simulink model "OLD_bidirection_buck_boost"  (R2025a)
settings: Solver=VariableStepAuto  StartTime=0.0  StopTime=0.1  MaxStep=1e-7  RelTol=1e-3
libraries: spsMosfetLib x5, spsPWMGeneratorDCDCLib x4, spsSeriesRLCBranchLib x4, spsCurrentMeasurementLib x3, spsVoltageMeasurementLib x2, spsDCVoltageSourceLib x1, spsGroundLib x1, spsMeanLib x1, spsPVArrayLib x1, spspowerguiLib x1
settings Model: Creator=GNKRISHNAN  LastModifiedBy=GNKRISHNAN

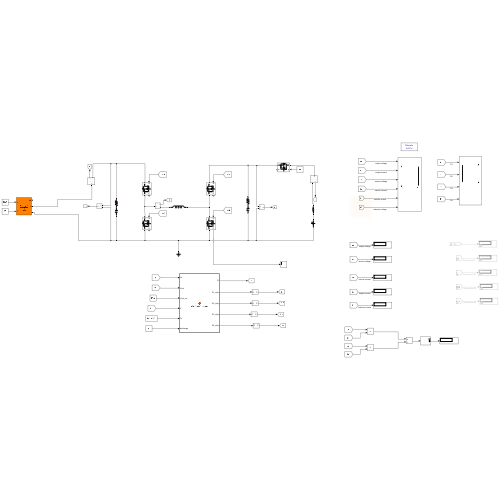
[thumbnail: Simulink's stored preview of the top-level diagram]
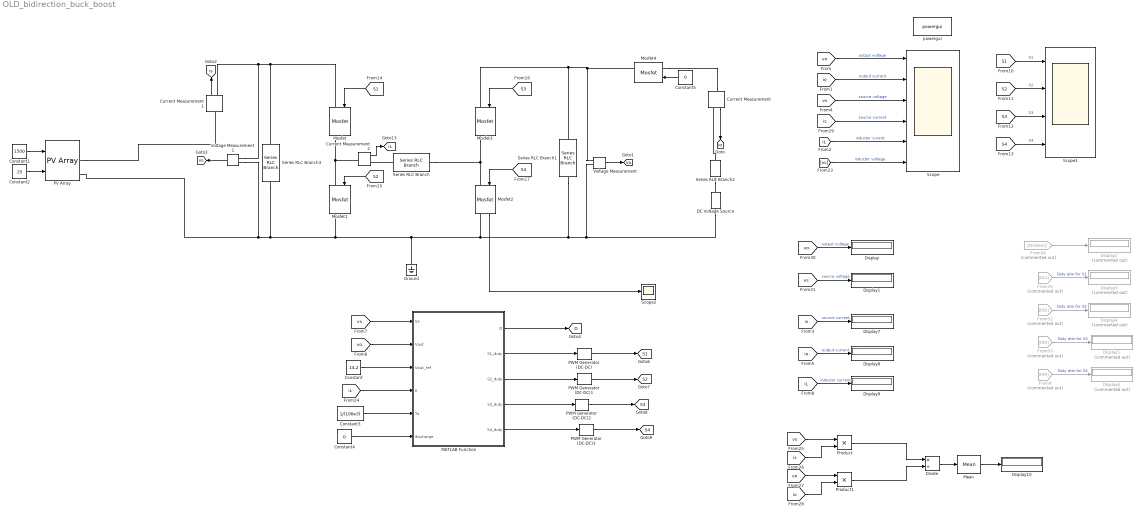
== system OLD_bidirection_buck_boost ==
  Constant : Constant  Value=14.2
  Constant1 : Constant  Value=1500
  Constant2 : Constant  Value=25
  Constant3 : Constant  Value=1/(100e3)
  Constant4 : Constant  Value=0
  Constant5 : Constant  Value=0
  Current Measurement : spsCurrentMeasurementLib/Current Measurement  PhasorSimulation=off  OutputType=Complex  PSBequivalent=0
  Current Measurement1 : spsCurrentMeasurementLib/Current Measurement  PhasorSimulation=off  OutputType=Complex  PSBequivalent=0
  Current Measurement2 : spsCurrentMeasurementLib/Current Measurement  PhasorSimulation=off  OutputType=Complex  PSBequivalent=0
  DC Voltage Source : spsDCVoltageSourceLib/DC Voltage Source  Amplitude=12  Measurements=None
  Display{,1,7..10} (6 alike) : Display
  Display{2..6} (5 alike) : Display  Commented=on
  Divide : Product  Inputs=*/
  From32 : From  Commented=on  GotoTag=DS2  TagVisibility=global
  From33 : From  Commented=on  GotoTag=DS3  TagVisibility=global
  From34 : From  Commented=on  GotoTag=Dintern  TagVisibility=global
  From35 : From  Commented=on  GotoTag=DS1  TagVisibility=global
  From9 : From  Commented=on  GotoTag=DS4  TagVisibility=global
  Ground : spsGroundLib/Ground  LConnTagsString=a
  MATLAB Function : MATLAB Function  TreatAsAtomicUnit=on  SystemSampleTime=1/(100e3)
  Mean : spsMeanLib/Mean  Freq=1/100e3  Vinit=0  Ts=0
  Mosfet{,1..3} (4 alike) : spsMosfetLib/Mosfet  Ron=0.1  Lon=0  Rd=0.0028  Vfd=0.7  IC=0  Rs=1e5  Cs=inf  Measurements=on
  Mosfet4 : spsMosfetLib/Mosfet  Ron=0.1  Lon=0  Rd=0.01  Vfd=0  IC=0  Rs=1e5  Cs=inf  Measurements=on
  PV Array : spsPVArrayLib/PV Array  Npar=1  Nser=1  PlotType=one module @ 25 deg.C & specified irradiances  S_vec="[ 1000  500  100 ]"  Temp_C_vec="[ 45 25  ]"  ModuleName=GCL System Integration Technology Co._ Ltd. GCL-P6/72355  PlotWhenSelected=off  Pm=355.0151  Ncell=72  Voc=47.9  Isc=9.74  Vm=39.49  Im=8.99  beta_Voc_pc=-0.296  alpha_Isc_pc=0.041201  beta_Voc=-0.14178  alpha_Isc=0.004013  IL=9.7653  I0=2.744e-11  nI=0.97505  Rsh=121.7675  Rs=0.31609  RobustModel=off  RobustCellTemperature=313.3991  BAL=on  Tc=1e-6  Tfilter=5e-5
  PWM Generator (DC-DC){,1..3} (4 alike) : spsPWMGeneratorDCDCLib/PWM Generator (DC-DC)  Fsw=100e3  Ts=0
  Product : Product
  Product1 : Product
  Scope : Scope  NumInputPorts=6
      settings: ActiveDisplayYMinimum=-1.5008435166057172  ActiveDisplayYMaximum=13.509037415165276
  Scope1 : Scope  NumInputPorts=4
      settings: ActiveDisplayYMinimum=-0.12499999999999997  ActiveDisplayYMaximum=1.125
  Scope2 : Scope
      settings: ActiveDisplayYMinimum=-1.430223431644835  ActiveDisplayYMaximum=12.872010884803517  DataLoggingVariableName=ScopeData2
  Series RLC Branch : spsSeriesRLCBranchLib/Series RLC Branch  LConnTagsString=__new0  RConnTagsString=__new0  BranchType=L  Resistance=0.001  Inductance=150e-6  SetiL0=on  InitialCurrent=0  Capacitance=1e-6  Setx0=off  InitialVoltage=0  Measurements=None
  Series RLC Branch1 : spsSeriesRLCBranchLib/Series RLC Branch  LConnTagsString=__new0  RConnTagsString=__new0  BranchType=RC  Resistance=0.0001  Inductance=1e-3  SetiL0=off  InitialCurrent=0  Capacitance=100e-6  Setx0=on  InitialVoltage=0  Measurements=None
  Series RLC Branch2 : spsSeriesRLCBranchLib/Series RLC Branch  LConnTagsString=__new0  RConnTagsString=__new0  BranchType=R  Resistance=83e-3  Inductance=1e-3  SetiL0=off  InitialCurrent=0  Capacitance=1e-6  Setx0=off  InitialVoltage=0  Measurements=None
  Series RLC Branch3 : spsSeriesRLCBranchLib/Series RLC Branch  LConnTagsString=__new0  RConnTagsString=__new0  BranchType=RC  Resistance=0.0001  Inductance=1e-3  SetiL0=off  InitialCurrent=0  Capacitance=100e-6  Setx0=on  InitialVoltage=0  Measurements=None
  Voltage Measurement : spsVoltageMeasurementLib/Voltage Measurement  PhasorSimulation=off  OutputType=Complex  PSBequivalent=0
  Voltage Measurement1 : spsVoltageMeasurementLib/Voltage Measurement  PhasorSimulation=off  OutputType=Complex  PSBequivalent=0
  powergui : spspowerguiLib/powergui  Priority=1  SimulationMode=Discrete  SampleTime=1e-7  frequency=60  Iterations=50  frequencyindice=0  Pbase=100e6  ErrMax=1e-4  UnitsV=kV  UnitsW=MW  buscounter=0  FunctionMessages=off  echomessages=off  EnableUseOfTLC=off  CurrentSourceSwitches=off  DisableSnubberDevices=off  DisableRonSwitches=off  DisableVfSwitches=off  DisplayEquations=off  AutomaticDiscreteSolvers=off  SolverType=Tustin/Backward Euler (TBE)  Interpol=off  ExternalGateDelay=off  methode=off  Ts=100  x0status=blocks  SPID=on  SwTol=0  HookPort=off  NonlinearTolerance=1e-4  nMaxIteration=100  ContinueOnMaxIteration=off  RestoreLinks=warning  ResistiveCurrentMeasurement=off  Frange=[0:2:500]  Ylog=off  Xlog=on  ShowGrid=off  save=off  variable=ZData  structure=0  ZoomFFT=off  StartTime=0.0  cycles=1  DisplayStyle=1  fundamental=60  FreqAxis=off  MaxFrequency=1000  frequencyindicesteady=1  RmsSteady=1  display=off
  tag scope: D=global, S1=global, S2=global, S3=global, S4=global, iL=global, io=global, is=global, vo=global, vs=global
  wires:
  [S1] -> Mosfet/1
  [S2] -> Mosfet1/1
  [S3] -> Mosfet3/1
  [S4] -> Mosfet2/1
  Voltage Measurement/1 -> [vo]
  Current Measurement/1 -> [io]
  Current Measurement1/1 -> [is]
  Voltage Measurement1/1 -> [vs]
  Constant1/1 -> PV Array/1
  Constant2/1 -> PV Array/2
  Mosfet2/1 -> Scope2/1
  MATLAB Function/5(S4_duty) -> PWM Generator (DC-DC)3/1
  PWM Generator (DC-DC)1/1 -> [S2]
  PWM Generator (DC-DC)2/1 -> [S3]
  PWM Generator (DC-DC)/1 -> [S1]
  MATLAB Function/4(S3_duty) -> PWM Generator (DC-DC)2/1
  MATLAB Function/1(D) -> [D]
  [vs] -> MATLAB Function/1(Vs)
  [vo] -> MATLAB Function/2(Vout)
  PWM Generator (DC-DC)3/1 -> [S4]
  Constant/1 -> MATLAB Function/3(Vout_ref)
  [iL] -> MATLAB Function/4(Il)
  Current Measurement2/1 -> [iL]
  Constant3/1 -> MATLAB Function/5(Ts)
  MATLAB Function/2(S1_duty) -> PWM Generator (DC-DC)/1
  MATLAB Function/3(S2_duty) -> PWM Generator (DC-DC)1/1
  Constant4/1 -> MATLAB Function/6(discharge)
  Constant5/1 -> Mosfet4/1
  [io] -> Display8/1  "output current"
  From32/1 -> Display4/1  "Duty atio for S2"
  From33/1 -> Display5/1  "Duty atio for S3"
  From35/1 -> Display3/1  "Duty atio for S1"
  From34/1 -> Display2/1
  [vo] -> Display/1  "output voltage"
  [vL] -> Scope/6  "inductor voltage"
  [vs] -> Display1/1  "source voltage"
  [is] -> Scope/4  "source current"
  [vo] -> Scope/1  "output voltage"
  Mean/1 -> Display10/1
  [is] -> Product/2
  [iL] -> Scope/5  "inductor curent"
  [vo] -> Product1/1
  [iL] -> Display9/1  "inductor current"
  [vs] -> Scope/3  "source voltage"
  Product1/1 -> Divide/2
  [vs] -> Product/1
  [S2] -> Scope1/2  "S2"
  [is] -> Display7/1  "source current"
  [S1] -> Scope1/1  "S1"
  Product/1 -> Divide/1
  Divide/1 -> Mean/1
  [io] -> Product1/2
  From9/1 -> Display6/1  "Duty atio for S4"
  [S4] -> Scope1/4  "S4"
  [io] -> Scope/2  "output current"
  [S3] -> Scope1/3  "S3"
  connections:
  Series RLC Branch/LConn1 -- Current Measurement2/RConn1
  Mosfet3/RConn1 -- Series RLC Branch/RConn1 -- Mosfet2/LConn1
  Series RLC Branch2/LConn1 -- Current Measurement/RConn1
  Series RLC Branch3/LConn1 -- Current Measurement1/RConn1 -- Voltage Measurement1/LConn1 -- Mosfet/LConn1
  PV Array/RConn1 -- Current Measurement1/LConn1
  Voltage Measurement/LConn2 -- DC Voltage Source/LConn1 -- Series RLC Branch1/RConn1 -- Mosfet2/RConn1 -- Mosfet1/RConn1 -- PV Array/RConn2 -- Voltage Measurement1/LConn2 -- Series RLC Branch3/RConn1 -- Ground/LConn1
  Current Measurement2/LConn1 -- Mosfet1/LConn1 -- Mosfet/RConn1
  Voltage Measurement/LConn1 -- Mosfet4/RConn1 -- Series RLC Branch1/LConn1 -- Mosfet3/LConn1
  Mosfet4/LConn1 -- Current Measurement/LConn1
  Series RLC Branch2/RConn1 -- DC Voltage Source/RConn1

== matlab function OLD_bidirection_buck_boost/MATLAB Function ==
  data: Vs input; D output; Vout input; Vout_ref input; Il input; S1_duty output; S2_duty output; S3_duty output; S4_duty output; Ts input; discharge input
function [D, S1_duty, S2_duty, S3_duty, S4_duty] = biDirBuckController(Vs, Vout, Vout_ref, Il, Ts, discharge)
% Codegen-safe digital controller for 4-switch bidirectional DC-DC
% Charge + Discharge
% - Charging branch: unchanged (original PI)
% - Discharge branch: uses mapping from spec (no switch swapping)
% - Sign-aware: during discharge Il < 0, controller drives negative Iref

% -------- Persistent declarations --------
persistent Kp_v Ki_v Kp_i Ki_i
persistent Dmax Il_max hyst
persistent v_int i_int Iref_min Iref_max

% Discharge-specific persistents
persistent Kp_v_d Ki_v_d Kp_i_d Ki_i_d
persistent v_int_d i_int_d
persistent Vref_dis Iref_dis_mag
persistent Dsmooth

% -------- Initialize persistents --------
if isempty(Kp_v)
    % Charge PI gains
    Kp_v = 0.4;   Ki_v = 60;
    Kp_i = 0.015; Ki_i = 150;
    
    % Limits
    Dmax     = 0.92;
    Il_max   = 3.0;
    hyst     = 0.5;
    Iref_min = 0.5;
    Iref_max = Il_max;
    
    % Charge integrators
    v_int = 0.0;  i_int = 0.0;
    
    % Discharge PI gains
    Kp_v_d = 0.7;   Ki_v_d = 100;
    Kp_i_d = 0.025; Ki_i_d = 250;
    v_int_d = 0.0;  i_int_d = 0.0;
    
    % Discharge refs
    Vref_dis     = 12.0;   % V
    Iref_dis_mag = 4.0;    % A (magnitude -> signed neg)
    
    % Duty smoothing
    Dsmooth = 0.0;
end

% -------- Default outputs --------
D       = 0.0;
S1_duty = 0.0;
S2_duty = 0.0;
S3_duty = 0.0;
S4_duty = 0.0;

% ============================================================
% -------- Discharge branch --------
if discharge == 1
    % Battery is Vout, DC bus is Vs
    batt_v = Vout;
    bus_v  = Vs;

    % Outer PI
    v_err_d = Vref_dis - batt_v;
    v_int_d = v_int_d + Ki_v_d * v_err_d * Ts;
    Iref_mag = v_int_d + Kp_v_d * v_err_d;
    
    if Iref_mag < 0, Iref_mag = 0; end
    if Iref_mag > Iref_dis_mag, Iref_mag = Iref_dis_mag; end
    
    Iref_d = -Iref_mag;   % discharge current reference (negative)
    
    % Inner PI (sign-aware)
    i_err_d = Il - Iref_d;
    i_int_d = i_int_d + Ki_i_d * i_err_d * Ts;
    u_p_d   = Kp_i_d * i_err_d;
    
    duty_raw = i_int_d + u_p_d;
    
    if duty_raw > Dmax
        D = Dmax;
        i_int_d = D - u_p_d;
    elseif duty_raw < 0
        D = 0.0;
        i_int_d = -u_p_d;
    else
        D = duty_raw;
    end
    
    % Smooth duty
    alpha = 0.01;
    Dsmooth = (1 - alpha) * Dsmooth + alpha * D;

    % -------- Region mapping (from spec) --------
    if bus_v > (batt_v + hyst)          % Boost mode
        % Q3=1, Q4=0, Q2=D, Q1=1-D
        S1_duty = 1 - Dsmooth;
        S2_duty = Dsmooth;
        S3_duty = 1.0;
        S4_duty = 0.0;

    elseif batt_v > (bus_v + hyst)      % Buck mode
        % Q1=1, Q2=0, Q3=D, Q4=1-D
        S1_duty = 1.0;
        S2_duty = 0.0;
        S3_duty = Dsmooth;
        S4_duty = 1 - Dsmooth;

    else                                % Buck-Boost mode
        % Q2=D, Q3=D, Q1=1-D, Q4=1-D
        S1_duty = 1 - Dsmooth;
        S2_duty = Dsmooth;
        S3_duty = Dsmooth;
        S4_duty = 1 - Dsmooth;
    end

    % -------- 6.4 Backup Mode --------
    % When DC Bus voltage > Battery Voltage
    % Q3=1, Q4=0, Q2=D, Q1=1-D -> synchronous boost converter
    if bus_v > batt_v
        S1_duty = 1 - Dsmooth;
        S2_duty = Dsmooth;
        S3_duty = 1.0;
        S4_duty = 0.0;
    end

else
% ============================================================
% -------- Charge branch (unchanged) --------
    if Vs > (Vout + hyst)
        region = 1; % Buck
    elseif abs(Vs - Vout) <= hyst
        region = 2; % Buck-Boost
    else
        region = 0; % Idle
    end

    % Voltage loop
    v_err = Vout_ref - Vout;
    v_int = v_int + Ki_v * v_err * Ts;
    Iref  = v_int + Kp_v * v_err;
    
    if Iref > Iref_max, Iref = Iref_max; end
    if Iref < Iref_min, Iref = Iref_min; end
    if Il >= Il_max, Iref = min(Iref, Il_max); end
    
    % Current loop
    i_err = Iref - Il;
    i_int = i_int + Ki_i * i_err * Ts;
    u_p   = Kp_i * i_err;
    
    duty_raw = i_int + u_p;
    
    if duty_raw > Dmax
        D = Dmax; i_int = D - u_p;
    elseif duty_raw < 0
        D = 0.0; i_int = -u_p;
    else
        D = duty_raw;
    end
    
    switch region
        case 1 % Buck
            S1_duty = D;
            S2_duty = 1 - D;
            S3_duty = 1.0;
            S4_duty = 0.0;
        case 2 % Buck-Boost
            S1_duty = D;
            S4_duty = D;
            S2_duty = 1 - D;
            S3_duty = 1 - D;
        otherwise % Idle
            S1_duty = 0.0;
            S2_duty = 0.0;
            S3_duty = 0.0;
            S4_duty = 0.0;
    end
end

% -------- Clamp duties --------
if S1_duty > 1, S1_duty = 1; elseif S1_duty < 0, S1_duty = 0; end
if S2_duty > 1, S2_duty = 1; elseif S2_duty < 0, S2_duty = 0; end
if S3_duty > 1, S3_duty = 1; elseif S3_duty < 0, S3_duty = 0; end
if S4_duty > 1, S4_duty = 1; elseif S4_duty < 0, S4_duty = 0; end

end
